simulink model "SIM"  (R2024b)
settings: Solver=VariableStepAuto  StartTime=0.0  StopTime=T  RelTol=1e-3
values from neighbouring files (symbols this model uses):
  A = [A zeros(5,1) ... (first row only)    [main.m]
  A_aug = [A zeros(5,1) ... (first row only)    [main_sim.m]
  ALPHA_MAX = 90 * pi/180    (= 1.57079632679)    [IP_MACRO.m]    (also in main_sim.m)
  B = [B ... (first row only)    [main.m]
  B_aug = [B; 0]    [main_sim.m]
  BETA_MAX = 15 * pi/180    (= 0.261799387799)    [IP_MACRO.m]    (also in main_sim.m)
  C = [C 0]    [main.m]
  C_aug = [C zeros(2,1)]    [main_sim.m]
  D = [0 0]'    [main.m]
  dead_zone_half_width = 0.2    [main_sim.m]
  K = lqr(A, B, Qr, Rr)    [IP_MACRO.m]    (also in main_sim.m = lqr(A_aug, B_aug, Qr, Rr))
  L_aug = [L ... (first row only)    [main_sim.m]
  noise_power = quant^2 / 12    (= 1.96091421467e-07)    [main_sim.m]
  noise_sample_time = 0.01    [main_sim.m]
  tau = 0.01    [main_sim.m]
  V_MAX = 5    [IP_MACRO.m]    (also in main_sim.m)
  V_MIN = -5    [IP_MACRO.m]    (also in main_sim.m)
  x0 = [0.1 0 0 0 0]'    [main.m]    (also in main_sim.m = [alpha_init 0 beta_init 0 0])
libraries: simulink_extras x1, simulink x1
settings Model: Creator=pedro  LastModifiedBy=pedro

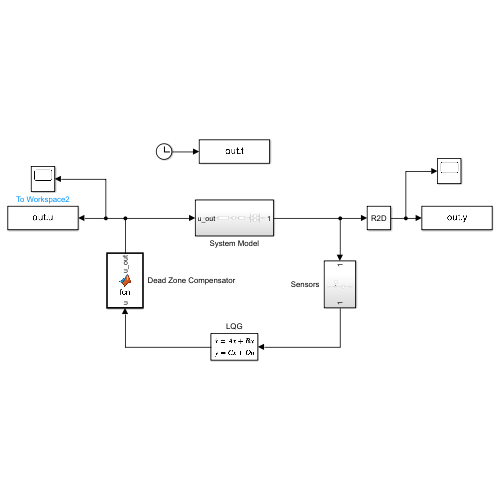
[thumbnail: Simulink's stored preview of the top-level diagram]
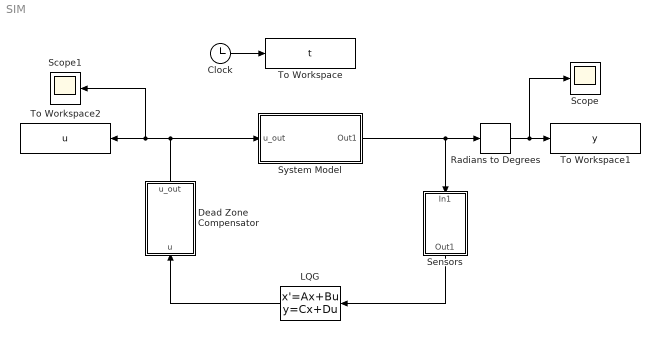
== system SIM ==
  Clock : Clock
  Dead Zone Compensator : MATLAB Function  TreatAsAtomicUnit=on
  LQG : StateSpace  A=A_aug - B_aug * K - L_aug * C_aug  B=L_aug  C=-K  D=zeros(1,2)  InitialCondition=zeros(6,1)
  Radians to Degrees : simulink_extras/Transformations/Radians to Degrees
  Scope : Scope
  Scope1 : Scope
  Sensors : Subsystem
  System Model : Subsystem
  To Workspace : ToWorkspace  VariableName=t  SaveFormat=Structure With Time  SampleTime=-1
  To Workspace1 : ToWorkspace  VariableName=y  SaveFormat=Structure With Time  SampleTime=-1
  To Workspace2 : ToWorkspace  VariableName=u  SaveFormat=Structure With Time  SampleTime=-1
  wires:
  Clock/1 -> To Workspace/1
  Radians to Degrees/1 -> Scope/1, To Workspace1/1
  System Model/1(Out1) -> Sensors/1(In1), Radians to Degrees/1
  LQG/1 -> Dead Zone Compensator/1(u)
  Dead Zone Compensator/1(u_out) -> System Model/1(u_out), Scope1/1, To Workspace2/1
  Sensors/1(Out1) -> LQG/1

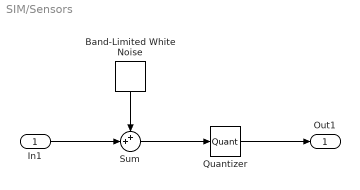
== system SIM/Sensors ==
  In1 : Inport
  Band-Limited White Noise : simulink/Sources/Band-Limited White Noise  Cov=[noise_power]  Ts=noise_sample_time  seed=[23341]
  Quantizer : Quantizer  QuantizationInterval=quant
  Sum : Sum  Inputs=++|
  Out1 : Outport
  wires:
  Sum/1 -> Quantizer/1
  Quantizer/1 -> Out1/1
  In1/1 -> Sum/2
  Band-Limited White Noise/1 -> Sum/1

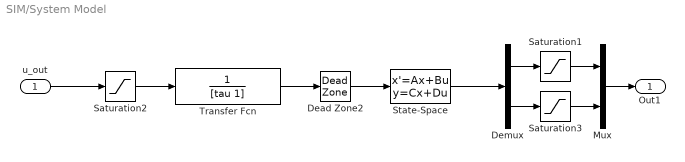
== system SIM/System Model ==
  u_out : Inport
  Dead Zone2 : DeadZone  LowerValue=-dead_zone_half_width  UpperValue=dead_zone_half_width
  Demux : Demux  Outputs=2
  Mux : Mux  Inputs=2
  Saturation1 : Saturate  UpperLimit=ALPHA_MAX  LowerLimit=-ALPHA_MAX
  Saturation2 : Saturate  UpperLimit=V_MAX  LowerLimit=V_MIN
  Saturation3 : Saturate  UpperLimit=BETA_MAX  LowerLimit=-BETA_MAX
  State-Space : StateSpace  A=A  B=B  C=C  D=D  InitialCondition=x0
  Transfer Fcn : TransferFcn  Denominator=[tau 1]
  Out1 : Outport
  wires:
  State-Space/1 -> Demux/1
  Demux/1 -> Saturation1/1
  Demux/2 -> Saturation3/1
  Saturation1/1 -> Mux/1
  Saturation3/1 -> Mux/2
  Mux/1 -> Out1/1
  u_out/1 -> Saturation2/1
  Dead Zone2/1 -> State-Space/1
  Saturation2/1 -> Transfer Fcn/1
  Transfer Fcn/1 -> Dead Zone2/1

== matlab function SIM/Dead Zone Compensator ==
  data: u input; u_out output
function u_out = fcn(u) 
    if u>0
        u_out= u + 0.2;
    elseif u<0
        u_out= u - 0.2;
    else 
        u_out = u;
    end
end
